simulink model "UDP_X_Plane_17_x_plane9"  (Simulink 7.8)
settings: Solver=ode45  StartTime=0.0  StopTime=inf  RelTol=1e-3
libraries: simulink x10, etargetslib x2, dspnetwork x2
settings Model: Creator=Andrey  LastModifiedBy=Andrey

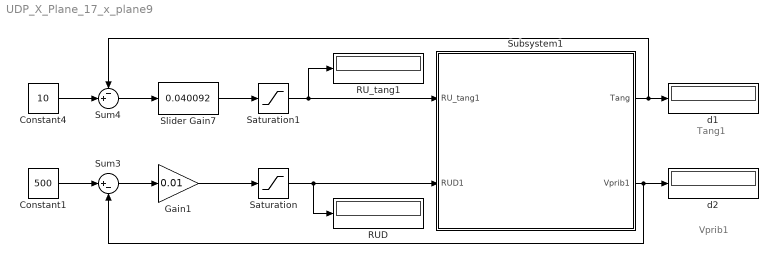
== system UDP_X_Plane_17_x_plane9 ==
  note: Tang1
  note: Vprib1
  Constant1 : Constant  Value=500  OutDataTypeStr=single  LockScale=on
  Constant4 : Constant  Value=10  OutDataTypeStr=single  LockScale=on
  Gain1 : Gain  Gain=0.01
  RUD : Display
  RU_tang1 : Display
  Saturation : Saturate  UpperLimit=1  LowerLimit=0
  Saturation1 : Saturate  UpperLimit=1  LowerLimit=-1
  Slider Gain7 : simulink/Math Operations/Slider Gain  low=-0.1  gain=0.040092  high=0.1
  Subsystem1 : Subsystem
  Sum3 : Sum  Inputs=|+-
  Sum4 : Sum  Inputs=-+|
  d1 : Display
  d2 : Display
  wires:
  Sum3/1 -> Gain1/1
  Subsystem1/1(Tang) -> d1/1, Sum4/1
  Gain1/1 -> Saturation/1
  Saturation1/1 -> Subsystem1/1(RU_tang1), RU_tang1/1
  Constant1/1 -> Sum3/1
  Slider Gain7/1 -> Saturation1/1
  Subsystem1/2(Vprib1) -> d2/1, Sum3/2
  Saturation/1 -> Subsystem1/2(RUD1), RUD/1
  Sum4/1 -> Slider Gain7/1
  Constant4/1 -> Sum4/2

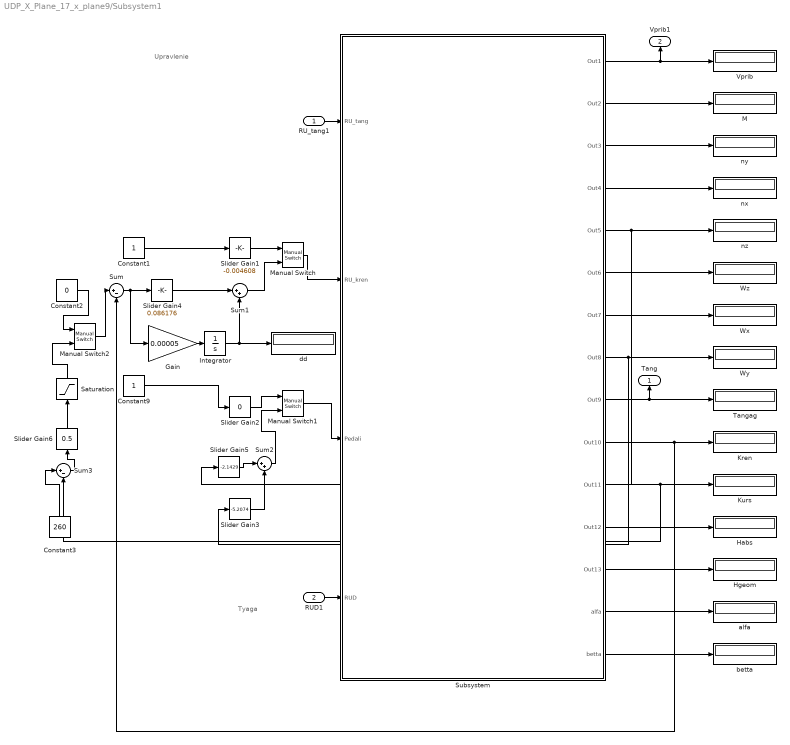
== system UDP_X_Plane_17_x_plane9/Subsystem1 ==
  note: Tyaga
  note: Upravlenie
  RU_tang1 : Inport
  RUD1 : Inport  Port=2
  Constant1 : Constant  OutDataTypeStr=single  LockScale=on
  Constant2 : Constant  Value=0  OutDataTypeStr=single  LockScale=on
  Constant3 : Constant  Value=260  OutDataTypeStr=single  LockScale=on
  Constant9 : Constant  OutDataTypeStr=single  LockScale=on
  Gain : Gain  Gain=0.00005
  Habs : Display
  Hgeom : Display
  Integrator : Integrator  LimitOutput=on  UpperSaturationLimit=1  LowerSaturationLimit=-1
  Kren : Display
  Kurs : Display
  M : Display
  Manual Switch : simulink/Signal Routing/Manual Switch  sw=0  action=0  varsize=off
  Manual Switch1 : simulink/Signal Routing/Manual Switch  sw=1  action=0  varsize=off
  Manual Switch2 : simulink/Signal Routing/Manual Switch  sw=1  action=0  varsize=off
  Saturation : Saturate  UpperLimit=45  LowerLimit=-45
  Slider Gain1 : simulink/Math Operations/Slider Gain  low=-1  gain=-0.004608  high=1
  Slider Gain2 : simulink/Math Operations/Slider Gain  low=-1  gain=0  high=1
  Slider Gain3 : simulink/Math Operations/Slider Gain  low=-10  gain=-5.2074  high=10
  Slider Gain4 : simulink/Math Operations/Slider Gain  low=-1.1  gain=0.086176  high=1.1
  Slider Gain5 : simulink/Math Operations/Slider Gain  low=-3  gain=-2.1429  high=3
  Slider Gain6 : simulink/Math Operations/Slider Gain  low=-1  gain=0.5  high=1
  Subsystem : Subsystem
  Sum : Sum  Inputs=|+-
  Sum1 : Sum  Inputs=|++
  Sum2 : Sum  Inputs=|++
  Sum3 : Sum  Inputs=|+-
  Tangag : Display
  Vprib : Display
  Wx : Display
  Wy : Display
  Wz : Display
  alfa : Display
  betta : Display
  dd : Display
  nx : Display
  ny : Display
  nz : Display
  Tang : Outport
  Vprib1 : Outport  Port=2
  wires:
  Subsystem/10(Out10) -> Sum/2, Kren/1
  Subsystem/11(Out11) -> Kurs/1, Sum3/2
  Constant9/1 -> Slider Gain2/1
  Subsystem/13(Out13) -> Hgeom/1
  Subsystem/12(Out12) -> Habs/1
  Subsystem/6(Out6) -> Wz/1
  Subsystem/7(Out7) -> Wx/1
  Subsystem/8(Out8) -> Wy/1, Slider Gain3/1
  Subsystem/2(Out2) -> M/1
  Subsystem/5(Out5) -> nz/1, Slider Gain5/1
  Subsystem/4(Out4) -> nx/1
  Subsystem/3(Out3) -> ny/1
  Subsystem/1(Out1) -> Vprib/1, Vprib1/1
  Constant1/1 -> Slider Gain1/1
  Subsystem/9(Out9) -> Tangag/1, Tang/1
  Manual Switch/1 -> Subsystem/2(RU_kren)
  Slider Gain1/1 -> Manual Switch/1
  Sum/1 -> Slider Gain4/1, Gain/1
  Slider Gain4/1 -> Sum1/1
  Sum1/1 -> Manual Switch/2
  Integrator/1 -> dd/1, Sum1/2
  Gain/1 -> Integrator/1
  Subsystem/14(alfa) -> alfa/1
  Subsystem/15(betta) -> betta/1
  RU_tang1/1 -> Subsystem/1(RU_tang)
  RUD1/1 -> Subsystem/4(RUD)
  Manual Switch1/1 -> Subsystem/3(Pedali)
  Slider Gain2/1 -> Manual Switch1/1
  Sum2/1 -> Manual Switch1/2
  Slider Gain5/1 -> Sum2/1
  Slider Gain3/1 -> Sum2/2
  Constant2/1 -> Manual Switch2/1
  Manual Switch2/1 -> Sum/1
  Constant3/1 -> Sum3/1
  Sum3/1 -> Slider Gain6/1
  Slider Gain6/1 -> Saturation/1
  Saturation/1 -> Manual Switch2/2

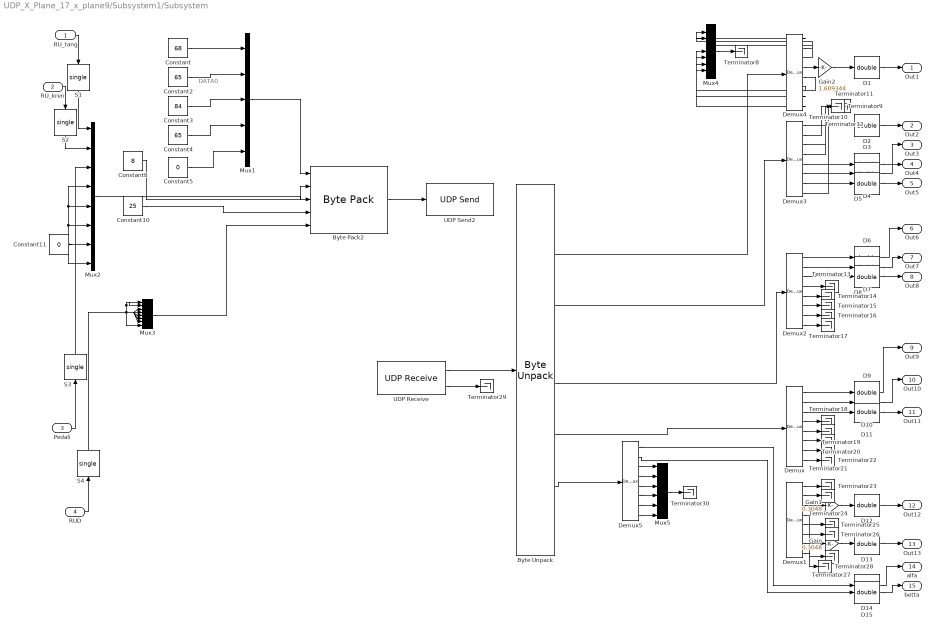
== system UDP_X_Plane_17_x_plane9/Subsystem1/Subsystem ==
  note: DATA0
  RU_tang : Inport
  RU_kren : Inport  Port=2
  Pedali : Inport  Port=3
  RUD : Inport  Port=4
  Byte Pack2 : etargetslib/Byte Pack  datatypes={'int8','int32','single','int32','single'}  byteAlign=1
  Byte Unpack : etargetslib/Byte Unpack  dimensions={[5+3*36],[1],[8],[1],[8],[12*36],[1],[8],[1],[8],[1],[8],[1],[8]}  datatypes={'int8','int32','single','int32','single','int8','int32','single','int32','single','int32','single','int32','single'}  byteAlign=1
  Constant : Constant  Value=68  OutDataTypeStr=int8
  Constant10 : Constant  Value=25  OutDataTypeStr=int32  LockScale=on
  Constant11 : Constant  Value=0  OutDataTypeStr=single  LockScale=on
  Constant2 : Constant  Value=65  OutDataTypeStr=int8  LockScale=on
  Constant3 : Constant  Value=84  OutDataTypeStr=int8
  Constant4 : Constant  Value=65  OutDataTypeStr=int8  LockScale=on
  Constant5 : Constant  Value=0  OutDataTypeStr=int8  LockScale=on
  Constant8 : Constant  Value=8  OutDataTypeStr=int32  LockScale=on
  D{1..15} (15 alike) : DataTypeConversion  OutDataTypeStr=double
  Demux{,1..5} (6 alike) : Demux  Outputs=8
  Gain : Gain  Gain=0.3048
  Gain1 : Gain  Gain=0.3048
  Gain2 : Gain  Gain=1.609344
  Mux1 : Mux  Inputs=5
  Mux2 : Mux  Inputs=8
  Mux3 : Mux  Inputs=8
  Mux4 : Mux  Inputs=7
  Mux5 : Mux  Inputs=6
  S{1..4} (4 alike) : DataTypeConversion  OutDataTypeStr=single
  Terminator{8..30} (23 alike) : Terminator
  UDP Receive : dspnetwork/UDP Receive  localURL='0.0.0.0'  localPort=4444  remoteURL='127.0.0.1'  remotePort=-1  recvBufferSize=8192  dims=720+5+36  signalDatatype=uint8  isVarSize=off  showBlockingTime=off  blockingTime=0  sampletime=inf
  UDP Send2 : dspnetwork/UDP Send  remoteURL='127.0.0.1'  remotePort=49000  localURL='0.0.0.0'  localPortSource=Automatically determine  localPort=4444  sampletime=-1  separateLengthPort=0
  Out1 : Outport
  Out2 : Outport  Port=2
  Out3 : Outport  Port=3
  Out4 : Outport  Port=4
  Out5 : Outport  Port=5
  Out6 : Outport  Port=6
  Out7 : Outport  Port=7
  Out8 : Outport  Port=8
  Out9 : Outport  Port=9
  Out10 : Outport  Port=10
  Out11 : Outport  Port=11
  Out12 : Outport  Port=12
  Out13 : Outport  Port=13
  alfa : Outport  Port=14
  betta : Outport  Port=15
  wires:
  Constant/1 -> Mux1/1
  Constant2/1 -> Mux1/2
  Constant3/1 -> Mux1/3
  Constant4/1 -> Mux1/4
  Constant5/1 -> Mux1/5
  Mux1/1 -> Byte Pack2/1
  Byte Pack2/1 -> UDP Send2/1
  Constant8/1 -> Byte Pack2/2
  Mux2/1 -> Byte Pack2/3
  Demux1/4 -> Gain/1
  Demux1/3 -> Gain1/1
  Byte Unpack/8 -> Demux2/1
  Byte Unpack/5 -> Demux3/1
  Demux4/4 -> Gain2/1
  Byte Unpack/3 -> Demux4/1
  RUD/1 -> S4/1
  Demux4/1 -> Mux4/1
  Demux4/2 -> Mux4/2
  Demux4/3 -> Mux4/3
  Demux4/5 -> Mux4/4
  Demux4/6 -> Mux4/5
  Demux4/7 -> Mux4/6
  Demux4/8 -> Mux4/7
  Mux4/1 -> Terminator8/1
  Demux3/2 -> Terminator9/1
  Demux3/3 -> Terminator10/1
  Demux3/4 -> Terminator11/1
  Demux3/8 -> Terminator12/1
  Demux2/4 -> Terminator13/1
  Demux2/5 -> Terminator14/1
  Demux2/6 -> Terminator15/1
  Demux2/7 -> Terminator16/1
  Demux2/8 -> Terminator17/1
  Demux/4 -> Terminator18/1
  Demux/5 -> Terminator19/1
  Demux/6 -> Terminator20/1
  Demux/7 -> Terminator21/1
  Demux/8 -> Terminator22/1
  Demux1/1 -> Terminator23/1
  Demux1/2 -> Terminator24/1
  Demux1/5 -> Terminator25/1
  Demux1/6 -> Terminator26/1
  Demux1/7 -> Terminator27/1
  Demux1/8 -> Terminator28/1
  Constant11/1 -> Mux2/4, Mux2/5, Mux2/6, Mux2/7, Mux2/8
  UDP Receive/2 -> Terminator29/1
  Gain2/1 -> D1/1
  Demux3/1 -> D2/1
  RU_tang/1 -> S1/1
  RU_kren/1 -> S2/1
  Demux3/5 -> D3/1
  Pedali/1 -> S3/1
  Demux3/6 -> D4/1
  Demux3/7 -> D5/1
  Demux2/1 -> D6/1
  Demux2/2 -> D7/1
  Demux2/3 -> D8/1
  Demux/1 -> D9/1
  Demux/2 -> D10/1
  Demux/3 -> D11/1
  Gain1/1 -> D12/1
  Gain/1 -> D13/1
  D1/1 -> Out1/1
  D2/1 -> Out2/1
  D3/1 -> Out3/1
  D4/1 -> Out4/1
  D5/1 -> Out5/1
  D6/1 -> Out6/1
  D7/1 -> Out7/1
  D8/1 -> Out8/1
  D9/1 -> Out9/1
  D10/1 -> Out10/1
  D11/1 -> Out11/1
  D12/1 -> Out12/1
  D13/1 -> Out13/1
  S1/1 -> Mux2/1
  S2/1 -> Mux2/2
  S3/1 -> Mux2/3
  S4/1 -> Mux3/8, Mux3/7, Mux3/6, Mux3/5, Mux3/4, Mux3/3, Mux3/2, Mux3/1
  Byte Unpack/12 -> Demux5/1
  Demux5/1 -> D14/1
  Demux5/2 -> D15/1
  Demux5/3 -> Mux5/1
  Demux5/4 -> Mux5/2
  Demux5/5 -> Mux5/3
  Demux5/6 -> Mux5/4
  Demux5/7 -> Mux5/5
  Demux5/8 -> Mux5/6
  Mux5/1 -> Terminator30/1
  D14/1 -> alfa/1
  D15/1 -> betta/1
  Constant10/1 -> Byte Pack2/4
  Mux3/1 -> Byte Pack2/5
  UDP Receive/1 -> Byte Unpack/1
  Byte Unpack/10 -> Demux/1
